simulink model "quadrotor_model_submission"  (R2019a)
settings: Solver=VariableStepAuto  StartTime=0.0  StopTime=10.0  RelTol=1e-3
undefined symbols (not defined in the file): g, K, m, sensor_noise_variance, x0
settings Model: Creator=tmcnama2  LastModifiedBy=tmcnama2
settings DataIOCC: InitialState=x0  LoadInitialState=on
settings DebuggingCC: InitInArrayFormatMsg=none

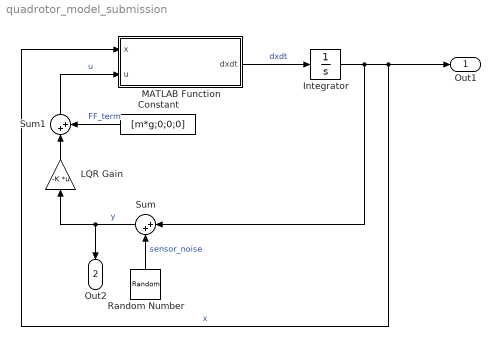
== system quadrotor_model_submission ==
  Constant : Constant  Value=[m*g;0;0;0]  VectorParams1D=off
  Integrator : Integrator  InitialCondition=x0
  "LQR Gain " : Gain  Gain=-K  Multiplication=Matrix(K*u)
  MATLAB Function : MATLAB Function  TreatAsAtomicUnit=on
  Random Number : RandomNumber  Mean=zeros(12,1)  Variance=sensor_noise_variance  SampleTime=0.1  VectorParams1D=off
  Sum : Sum  Inputs=|++
  Sum1 : Sum  Inputs=|++
  Out1 : Outport  SignalName=x
  Out2 : Outport  Port=2  SignalName=y
  wires:
  MATLAB Function/1(dxdt) -> Integrator/1  "dxdt"
  Integrator/1 -> Out1/1, MATLAB Function/1(x), Sum/1  "x"
  Random Number/1 -> Sum/2  "sensor_noise"
  Sum/1 -> Out2/1, "LQR Gain "/1  "y"
  Sum1/1 -> MATLAB Function/2(u)  "u"
  "LQR Gain "/1 -> Sum1/1
  Constant/1 -> Sum1/2  "FF_term"

== matlab function quadrotor_model_submission/MATLAB Function ==
  data: x input; u input; dxdt output
function dxdt = quadrotor_dynamics(x, u)
    m = 0.6;
    Jx = 0.0092;
    Jy = 0.0091;
    Jz = 0.0101;
    g = 9.81;
    px_dot = x(1);
%   px =     x(2);
    py_dot = x(3);
%   py =     x(4);
    pz_dot = x(5);
%   pz =     x(6);
    p =      x(7);
    phi =    x(8);
    q =      x(9); 
    theta =  x(10);
    r =      x(11);
    psi =    x(12);
    
    u_clipped = zeros(4,1);
    u_clipped(1) = max([min([u(1), 16]),0]);
    u_clipped(2) = max([min([u(2), .432]),-.432]);
    u_clipped(3) = max([min([u(3), .432]),-.432]);
    u_clipped(4) = max([min([u(4), .1]),-.1]);
    
    F = u_clipped(1);
    tau_phi = u_clipped(2);
    tau_theta = u_clipped(3);
    tau_psi = u_clipped(4);
    
    az = -F/m;

    dxdt =  [cos(phi)*sin(theta)*az;
             px_dot;
             -sin(phi)*az;
             py_dot;
             g + cos(phi)*cos(theta)*az;
             pz_dot;             
             1/Jx*tau_phi;
             p + q*sin(phi)*tan(theta) + r*cos(phi)*tan(theta);
             1/Jy*tau_theta;
             q*cos(phi) - r*sin(phi);
             1/Jz*tau_psi;
             q*sin(phi)/cos(theta) + r*cos(phi)/cos(theta)];
